simulink model "models_multirate_data_example_2022b"  (R2022b)
settings: Solver=VariableStepAuto  StartTime=0.0  StopTime=StopTime  FixedStep=-1  RelTol=1e-4  AbsTol=1e-5
values from neighbouring files (symbols this model uses):
  Fs = 1024    [collabrative_aug_30.m]    (also in generate_test_data.m = 1000; multi_rate_cherry_may_16.m = 1/Ts; onesensor_with_less_batch_works_perfect_200.m; twosensor_onesensor_comparison_noisy.m)
  GG = tf(1, [20 1])    [collabrative_aug_30.m]    (also in onesensor_with_less_batch_works_perfect_200.m = tf(1, [1 3 1 1]); twosensor_onesensor_comparison_noisy.m = tf(1, [1 3 1 1]); validate_camera_ready_testn2.m = tf(num, den); validate_order_TC_peak.m = tf(num, den))
  m = 2    [collabrative_aug_30.m]    (also in multi_rate_cherry_may_16.m = 1; onesensor_with_less_batch_works_perfect_200.m; twosensor_onesensor_comparison_noisy.m; validate_camera_ready_testn2.m)
  n1 = 3    [collabrative_aug_30.m]    (also in multi_rate_cherry_may_16.m = 2; onesensor_with_less_batch_works_perfect_200.m; twosensor_onesensor_comparison_noisy.m = 5; validate_camera_ready_testn2.m)
  n2 = 5    [collabrative_aug_30.m]    (also in multi_rate_cherry_may_16.m = 3; onesensor_with_less_batch_works_perfect_200.m; twosensor_onesensor_comparison_noisy.m = 7; validate_camera_ready_testn2.m)
settings Model: Creator=tpjch  LastModifiedBy=31701
settings SolverCC: AutoScaleAbsTol=off
settings OptimizationCC: ReuseModelBlockBuffer=on

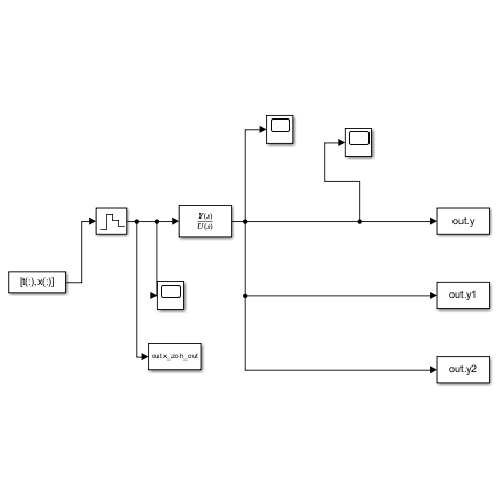
[thumbnail: Simulink's stored preview of the top-level diagram]
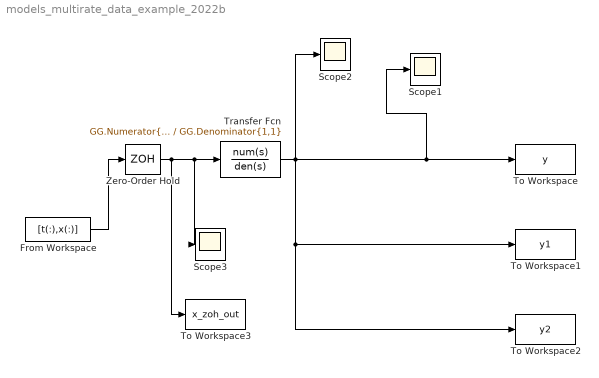
== system models_multirate_data_example_2022b ==
  From Workspace : FromWorkspace  VariableName=[t(:),x(:)]  OutDataTypeStr=double  SampleTime=1/Fs  Interpolate=off  ZeroCross=off  OutputAfterFinalValue=Holding final value
  Scope1 : Scope
  Scope2 : Scope
  Scope3 : Scope
  To Workspace : ToWorkspace  VariableName=y  SampleTime=1/Fs
  To Workspace1 : ToWorkspace  VariableName=y1  SampleTime=1/Fs*n1
  To Workspace2 : ToWorkspace  VariableName=y2  SampleTime=1/Fs*n2
  To Workspace3 : ToWorkspace  VariableName=x_zoh_out  SampleTime=1/Fs
  Transfer Fcn : TransferFcn  Numerator=GG.Numerator{1,1}  Denominator=GG.Denominator{1,1}
  Zero-Order Hold : ZeroOrderHold  SampleTime=1/Fs*m
  wires:
  Zero-Order Hold/1 -> To Workspace3/1, Scope3/1, Transfer Fcn/1
  From Workspace/1 -> Zero-Order Hold/1
  Transfer Fcn/1 -> To Workspace2/1, To Workspace1/1, To Workspace/1, Scope1/1, Scope2/1
